simulink model "openfast_validation_test"  (R2021a)
settings: Solver=ode4  StartTime=0.0  StopTime=TMax  FixedStep=DT  MaxStep=DT  RelTol=1e-3  EnableMultiTasking=on
undefined symbols (not defined in the file or in its folder): OutList, strmatch
settings Model: Creator=bjonkman  LastModifiedBy=cam
settings SolverCC: AlgebraicLoopSolver=TrustRegion
settings DataIOCC: LimitDataPoints=on  SaveFormat=Array  SaveOutput=off  SaveTime=off  ReturnWorkspaceOutputs=off  SignalLoggingName=sigsOut
settings OptimizationCC: ExpressionDepthLimit=2147483647  LifeSpan=inf
settings DebuggingCC: SaveWithParameterizedLinksMsg=none  UnderspecifiedInitializationDetection=Classic  MergeDetectMultiDrivingBlocksExec=none  SignalResolutionControl=TryResolveAllWithWarning  InheritedTsInSrcMsg=none  MultiTaskDSMMsg=warning  MultiTaskCondExecSysMsg=none  FcnCallInpInsideContextMsg=warning  StateNameClashWarn=warning  SFUnexpectedBacktrackingDiag=warning  SFNoUnconditionalDefaultTransitionDiag=warning  SFExecutionAtInitializationDiag=none  SFMachineParentedDataDiag=warning  ArithmeticOperatorsInVariantConditions=warning
settings HardwareCC: ProdBitPerPointer=32  ProdBitPerSizeT=32  ProdBitPerPtrDiffT=32  ProdLargestAtomicFloat=None  ProdIntDivRoundTo=Undefined  ProdEndianess=Unspecified  ProdWordSize=32  ProdHWDeviceType=32-bit Generic  TargetBitPerLong=64  TargetBitPerPointer=64  TargetBitPerSizeT=64  TargetBitPerPtrDiffT=64  TargetLongLongMode=on  TargetIntDivRoundTo=Zero  TargetEndianess=LittleEndian  TargetWordSize=64  TargetHWDeviceType=MATLAB Host  ProdEqTarget=off
settings ModelReferenceCC: PropagateSignalLabelsOutOfModel=off
settings SFSimCC: SimUseLocalCustomCode=off  CustomCodeUndefinedFunction=UseInterfaceOnly
settings RTWCC: RTWUseLocalCustomCode=off
settings CodeAppCC: StateflowObjectComments=on
settings GRTTargetCC: TargetLangStandard=C89/C90 (ANSI)  CombineOutputUpdateFcns=off  GRTInterface=on
settings ConfigComp: CovMetricSettings=dw  CovSaveCumulativeToWorkspaceVar=on  CovSaveSingleToWorkspaceVar=on  CovExternalEMLEnable=off

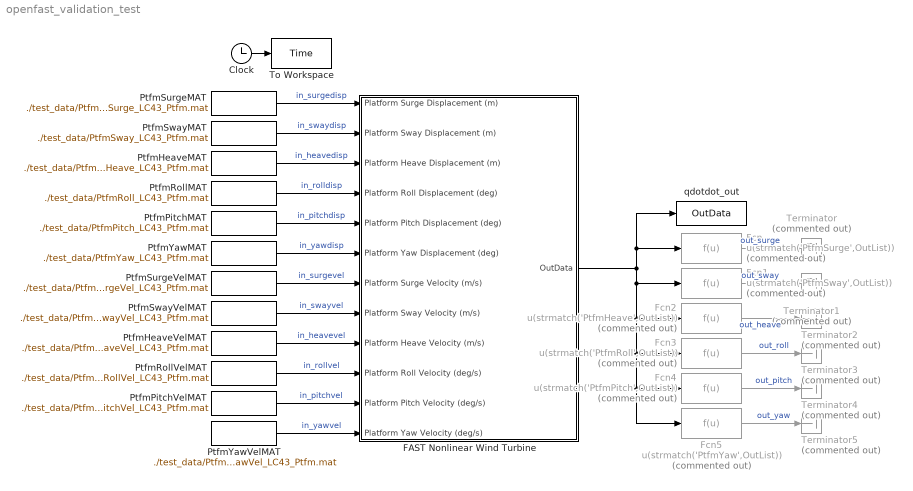
== system openfast_validation_test ==
  Clock : Clock
  FAST Nonlinear Wind Turbine : Subsystem  mask(FAST Nonlinear Wind Turbine){}
      mask help: This block contains the FAST S-Function.
      mask init:
      | clear FAST_SFunc
  Fcn : Fcn  Commented=on  Expr=u(strmatch('PtfmSurge',OutList))
  Fcn1 : Fcn  Commented=on  Expr=u(strmatch('PtfmSway',OutList))
  Fcn2 : Fcn  Commented=on  Expr=u(strmatch('PtfmHeave',OutList))
  Fcn3 : Fcn  Commented=on  Expr=u(strmatch('PtfmRoll',OutList))
  Fcn4 : Fcn  Commented=on  Expr=u(strmatch('PtfmPitch',OutList))
  Fcn5 : Fcn  Commented=on  Expr=u(strmatch('PtfmYaw',OutList))
  PtfmHeaveMAT : FromFile  FileName=./test_data/PtfmHeave_LC43_Ptfm.mat
  PtfmHeaveVelMAT : FromFile  FileName=./test_data/PtfmHeaveVel_LC43_Ptfm.mat
  PtfmPitchMAT : FromFile  FileName=./test_data/PtfmPitch_LC43_Ptfm.mat
  PtfmPitchVelMAT : FromFile  FileName=./test_data/PtfmPitchVel_LC43_Ptfm.mat
  PtfmRollMAT : FromFile  FileName=./test_data/PtfmRoll_LC43_Ptfm.mat
  PtfmRollVelMAT : FromFile  FileName=./test_data/PtfmRollVel_LC43_Ptfm.mat
  PtfmSurgeMAT : FromFile  FileName=./test_data/PtfmSurge_LC43_Ptfm.mat
  PtfmSurgeVelMAT : FromFile  FileName=./test_data/PtfmSurgeVel_LC43_Ptfm.mat
  PtfmSwayMAT : FromFile  FileName=./test_data/PtfmSway_LC43_Ptfm.mat
  PtfmSwayVelMAT : FromFile  FileName=./test_data/PtfmSwayVel_LC43_Ptfm.mat
  PtfmYawMAT : FromFile  FileName=./test_data/PtfmYaw_LC43_Ptfm.mat
  PtfmYawVelMAT : FromFile  FileName=./test_data/PtfmYawVel_LC43_Ptfm.mat
  Terminator{,1..5} (6 alike) : Terminator  Commented=on
  To Workspace : ToWorkspace  VariableName=Time  SampleTime=-1
  qdotdot_out : ToWorkspace  VariableName=OutData  SampleTime=-1
  wires:
  Clock/1 -> To Workspace/1
  PtfmSurgeMAT/1 -> FAST Nonlinear Wind Turbine/1(Platform Surge Displacement (m))  "in_surgedisp"
  PtfmYawMAT/1 -> FAST Nonlinear Wind Turbine/6(Platform Yaw Displacement (deg))  "in_yawdisp"
  PtfmPitchMAT/1 -> FAST Nonlinear Wind Turbine/5(Platform Pitch Displacement (deg))  "in_pitchdisp"
  PtfmRollMAT/1 -> FAST Nonlinear Wind Turbine/4(Platform Roll Displacement (deg))  "in_rolldisp"
  PtfmHeaveMAT/1 -> FAST Nonlinear Wind Turbine/3(Platform Heave Displacement (m))  "in_heavedisp"
  PtfmSwayMAT/1 -> FAST Nonlinear Wind Turbine/2(Platform Sway Displacement (m))  "in_swaydisp"
  FAST Nonlinear Wind Turbine/1(OutData) -> qdotdot_out/1, Fcn/1, Fcn5/1, Fcn4/1, Fcn3/1, Fcn2/1, Fcn1/1
  Fcn/1 -> Terminator/1  "out_surge"
  Fcn1/1 -> Terminator1/1  "out_sway"
  Fcn5/1 -> Terminator5/1  "out_yaw"
  Fcn4/1 -> Terminator4/1  "out_pitch"
  Fcn3/1 -> Terminator3/1  "out_roll"
  Fcn2/1 -> Terminator2/1  "out_heave"
  PtfmSwayVelMAT/1 -> FAST Nonlinear Wind Turbine/8(Platform Sway Velocity (m/s))  "in_swayvel"
  PtfmRollVelMAT/1 -> FAST Nonlinear Wind Turbine/10(Platform Roll Velocity (deg/s))  "in_rollvel"
  PtfmHeaveVelMAT/1 -> FAST Nonlinear Wind Turbine/9(Platform Heave Velocity (m/s))  "in_heavevel"
  PtfmYawVelMAT/1 -> FAST Nonlinear Wind Turbine/12(Platform Yaw Velocity (deg/s))  "in_yawvel"
  PtfmPitchVelMAT/1 -> FAST Nonlinear Wind Turbine/11(Platform Pitch Velocity (deg/s))  "in_pitchvel"
  PtfmSurgeVelMAT/1 -> FAST Nonlinear Wind Turbine/7(Platform Surge Velocity (m/s))  "in_surgevel"

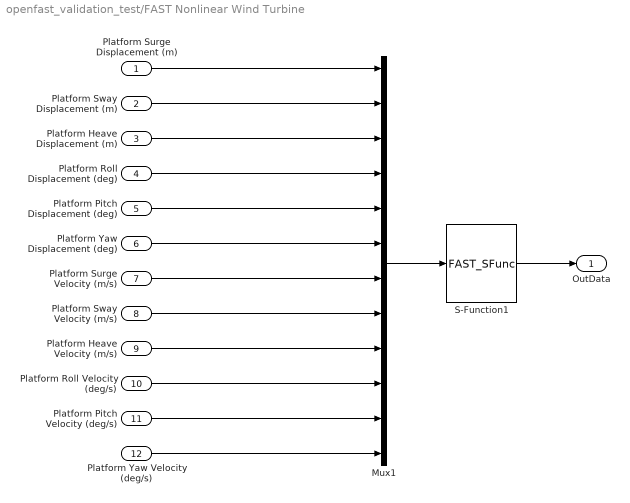
== system openfast_validation_test/FAST Nonlinear Wind Turbine ==
  Platform Surge Displacement (m) : Inport
  Platform Sway Displacement (m) : Inport  Port=2
  Platform Heave Displacement (m) : Inport  Port=3
  Platform Roll Displacement (deg) : Inport  Port=4
  Platform Pitch Displacement (deg) : Inport  Port=5
  Platform Yaw Displacement (deg) : Inport  Port=6
  Platform Surge Velocity (m/s) : Inport  Port=7
  Platform Sway Velocity (m/s) : Inport  Port=8
  Platform Heave Velocity (m/s) : Inport  Port=9
  Platform Roll Velocity (deg/s) : Inport  Port=10
  Platform Pitch Velocity (deg/s) : Inport  Port=11
  Platform Yaw Velocity (deg/s) : Inport  Port=12
  Mux1 : Mux  Inputs=12
  S-Function1 : S-Function  FunctionName=FAST_SFunc  Parameters=FAST_InputFileName, TMax, 0  SFunctionDeploymentMode=off  EnableBusSupport=off
  OutData : Outport
  wires:
  S-Function1/1 -> OutData/1
  Mux1/1 -> S-Function1/1
  Platform Surge Displacement (m)/1 -> Mux1/1
  Platform Sway Displacement (m)/1 -> Mux1/2
  Platform Heave Displacement (m)/1 -> Mux1/3
  Platform Roll Displacement (deg)/1 -> Mux1/4
  Platform Pitch Displacement (deg)/1 -> Mux1/5
  Platform Yaw Displacement (deg)/1 -> Mux1/6
  Platform Surge Velocity (m/s)/1 -> Mux1/7
  Platform Yaw Velocity (deg/s)/1 -> Mux1/12
  Platform Pitch Velocity (deg/s)/1 -> Mux1/11
  Platform Roll Velocity (deg/s)/1 -> Mux1/10
  Platform Heave Velocity (m/s)/1 -> Mux1/9
  Platform Sway Velocity (m/s)/1 -> Mux1/8
